simulink model "Task4_2"  (R2020b)
settings: Solver=VariableStepAuto  StartTime=0.0  StopTime=10.0  RelTol=1e-3
values from neighbouring files (symbols this model uses):
  Cp_opt = lambda_opt * Ct_opt    (= 0.4375971)    [Code2021_Jo_Saleh.m]    (also in ExeRet21.m.m)
  K = p * tau_z / (tau_pl * 2*we * tau_w)    (= -13.4008504823)    [Code2021_Jo_Saleh.m]    (also in ExeRet21.m.m)
  lambda_opt = 6.7    [Code2021_Jo_Saleh.m]    (also in ExeRet21.m.m)
  p = 180    [Code2021_Jo_Saleh.m]    (also in ExeRet21.m.m)
  r = 50    [Code2021_Jo_Saleh.m]    (also in ExeRet21.m.m)
  rho = 1.225    [Code2021_Jo_Saleh.m]    (also in ExeRet21.m.m)
  Rs = 60e-3    (= 0.06)    [Code2021_Jo_Saleh.m]    (also in ExeRet21.m.m)
  tau_le = tau_w    (= 8.82652066845)    [Code2021_Jo_Saleh.m]    (also in ExeRet21.m.m)
  tau_lg = tau_z    (= -109.330180381)    [Code2021_Jo_Saleh.m]    (also in ExeRet21.m.m)
  Te_rated = (Ptur * p) / (2 * we)    (= 1671126.90246)    [Code2021_Jo_Saleh.m]    (also in ExeRet21.m.m)
settings Model: Creator=Tomo  LastModifiedBy=Tomo

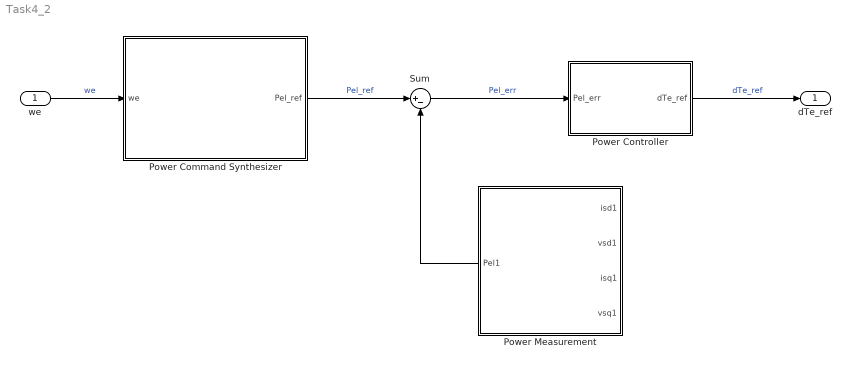
== system Task4_2 ==
  we : Inport
  Power Command Synthesizer : Subsystem
  Power Controller : Subsystem
  Power Measurement : Subsystem
  Sum : Sum  Inputs=|+-
  dTe_ref : Outport
  wires:
  we/1 -> Power Command Synthesizer/1(we)  "we"
  Power Command Synthesizer/1(Pel_ref) -> Sum/1  "Pel_ref"
  Sum/1 -> Power Controller/1(Pel_err)  "Pel_err"
  Power Measurement/1(Pel1) -> Sum/2
  Power Controller/1(dTe_ref) -> dTe_ref/1  "dTe_ref"

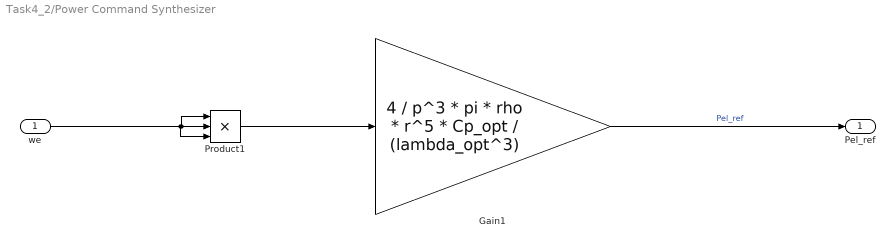
== system Task4_2/Power Command Synthesizer ==
  we : Inport
  Gain1 : Gain  Gain=4 / p^3 * pi * rho * r^5 * Cp_opt / (lambda_opt^3)
  Product1 : Product  Inputs=3
  Pel_ref : Outport
  wires:
  we/1 -> Product1/2, Product1/1, Product1/3
  Product1/1 -> Gain1/1
  Gain1/1 -> Pel_ref/1  "Pel_ref"

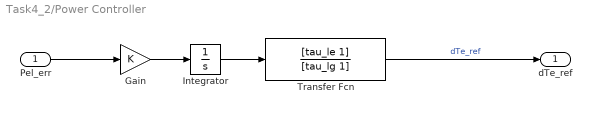
== system Task4_2/Power Controller ==
  Pel_err : Inport
  Gain : Gain  Gain=K
  Integrator : Integrator  InitialCondition=Te_rated
  Transfer Fcn : TransferFcn  Numerator=[tau_le 1]  Denominator=[tau_lg 1]
  dTe_ref : Outport
  wires:
  Transfer Fcn/1 -> dTe_ref/1  "dTe_ref"
  Gain/1 -> Integrator/1
  Integrator/1 -> Transfer Fcn/1
  Pel_err/1 -> Gain/1

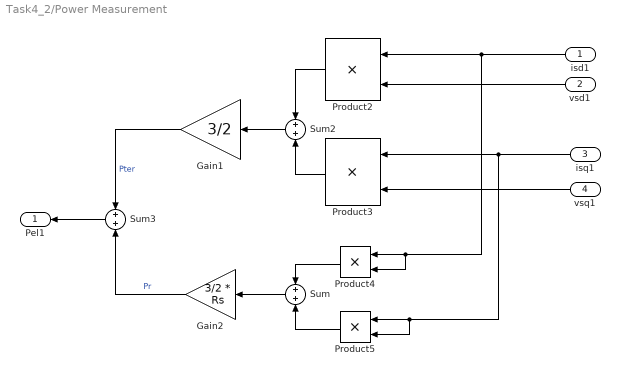
== system Task4_2/Power Measurement ==
  isd1 : Inport
  vsd1 : Inport  Port=2
  isq1 : Inport  Port=3
  vsq1 : Inport  Port=4
  Gain1 : Gain  Gain=3/2
  Gain2 : Gain  Gain=3/2 * Rs
  Product{2..5} (4 alike) : Product
  Sum : Sum  Inputs=+|+
  Sum2 : Sum  Inputs=+|+
  Sum3 : Sum  Inputs=+|+
  Pel1 : Outport
  wires:
  Sum/1 -> Gain2/1
  Product4/1 -> Sum/1
  Product5/1 -> Sum/2
  Sum3/1 -> Pel1/1
  Gain1/1 -> Sum3/1  "Pter"
  Product2/1 -> Sum2/1
  Product3/1 -> Sum2/2
  isd1/1 -> Product4/2, Product4/1, Product2/1
  vsd1/1 -> Product2/2
  vsq1/1 -> Product3/2
  Gain2/1 -> Sum3/2  "Pr"
  Sum2/1 -> Gain1/1
  isq1/1 -> Product5/2, Product5/1, Product3/1
